simulink model "FOC_Motor_Tuning"  (R2025b)
settings: Solver=VariableStepAuto  StartTime=0.0  StopTime=8  RelTol=1e-3
values from neighbouring files (symbols this model uses):
  adc : value not decoded    [FoCFpgaData.sldd]
  dataRange = 800.0    [FoCFpgaData.sldd]
  encoder = 0.0    [FoCFpgaData.sldd]
  inverter = 24.0    [FoCFpgaData.sldd]
  paramAdcAmperePerCount : value not decoded    [FoCFpgaData.sldd]
  paramAdcCalibrationSamples = 16.0    [FoCFpgaData.sldd]
  paramAdcCountAtZeroAmpere : value not decoded    [FoCFpgaData.sldd]
  paramAdcEnablecalibration = 1.0    [FoCFpgaData.sldd]
  paramCurrentControlSatVoltage = 13.856406460551021    [FoCFpgaData.sldd]
  paramEncoderCalibrationDuration = 0.2    [FoCFpgaData.sldd]
  paramEncoderCalibrationMaxError = 0.0012566370614359172    [FoCFpgaData.sldd]
  paramEncoderCalibrationVoltage = 2.0    [FoCFpgaData.sldd]
  paramEncoderRotorPositionAtZeroCount = 0.0    [FoCFpgaData.sldd]
  paramOpenLoopVelocityAcceleration = 40.0    [FoCFpgaData.sldd]
  paramOpenLoopVelocityToVoltsBias = 0.4    [FoCFpgaData.sldd]
  paramOpenLoopVelocityToVoltsScalar = 0.04    [FoCFpgaData.sldd]
  paramOverCurrentDuration = 0.05    [FoCFpgaData.sldd]
  paramOverCurrentEnable = 0.0    [FoCFpgaData.sldd]
  paramOverCurrentLimit = 10.45    [FoCFpgaData.sldd]
  paramPwmCompareAtZeroVolt = 500.0    [FoCFpgaData.sldd]
  paramPwmCompareMax = 1000.0    [FoCFpgaData.sldd]
  paramPwmComparePerVolt = 41.666666666666664    [FoCFpgaData.sldd]
  paramVelocityControlSatCurrent = 3.5    [FoCFpgaData.sldd]
  PI_params = 0.00048000000000000007    [FoCFpgaData.sldd]
  pmsm : value not decoded    [FoCFpgaData.sldd]
  pwm = 2.0E-8    [FoCFpgaData.sldd]
  sampleTime = 4.0E-5    [FoCFpgaData.sldd]
libraries: fl_lib x12, nesl_utility x12, mcbeeMathTransformLib x8, simulink x4, slpidlib x4, ee_lib x4, mcbpositiondecoderlib x3, mcbcontrolslib x3, mcbplantlib x1, autolibpmsmexterior x1, eeGeneralControl x1, SignalEditorBlockLib x1
(part 2 of 3)

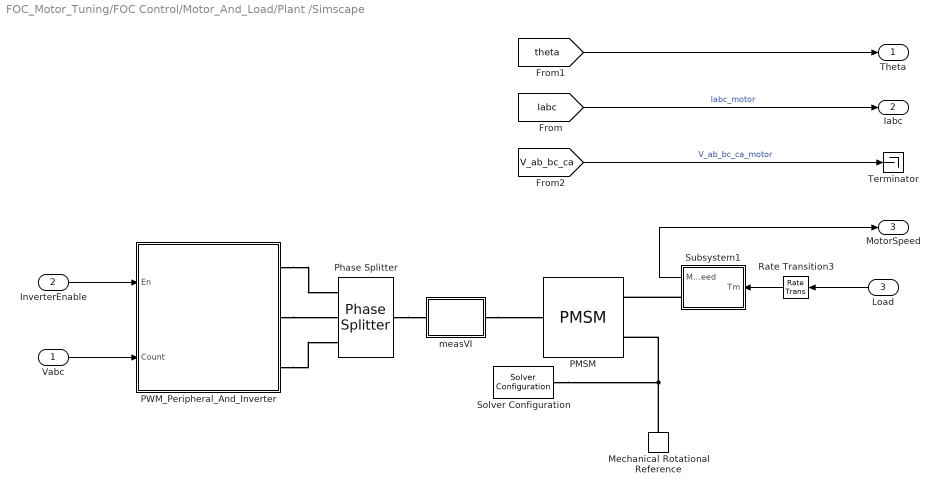
== system FOC_Motor_Tuning/FOC Control/Motor_And_Load/Plant /Simscape ==
  Vabc : Inport
  InverterEnable : Inport  Port=2
  Load : Inport  Port=3
  Mechanical Rotational Reference : fl_lib/Mechanical/Rotational Elements/Mechanical Rotational Reference
  PMSM : ee_lib/Electromechanical/Permanent Magnet/PMSM  port_option=ee.enum.threePhasePort.composite  winding_type=ee.enum.statorconnection.wye  machine_param=ee.enum.pmsm.parameterization.constant  nPolePairs=pmsm.p  pmflux_param=ee.enum.pmflux.fluxlinkage  pm_flux_linkage=pmsm.FluxPM Wb  torque_constant=0.18 N*m/A  back_emf_constant=0.18 V/(rad/s)  stator_param=ee.enum.statorparam.LdLqL0  Ld=pmsm.Ld H  Lq=pmsm.Lq H  idVec=[-200, 0, 200] A  iqVec=[-200, 0, 200] A  LdMatrix=0.0002 * ones(3, 3) H  LqMatrix=0.0002 * ones(3, 3) H  PmMatrix=0.1 * ones(3, 3) Wb  ktMatrix=0.18 * ones(3, 3) N*m/A  keMatrix=0.18 * ones(3, 3) V/(rad/s)  L0=0 H  Ls=0.0002 H  Lm=-0.00002 H  Ms=0.00002 H  Rs=pmsm.Rs Ohm  zero_sequence=ee.enum.park.zerosequence.exclude  axes_param=ee.enum.rotorangle.daxis  loss_param=ee.enum.ironloss.none  losses_oc=[0, 0, 0] W  losses_sc=[0, 0, 0] W  f_losses=60 Hz  Isc_losses=95 A  J=pmsm.J kg*m^2  lam=pmsm.B N*m/(rad/s)  i_d_specify=off  i_d_priority=None  i_d=0 A  i_d_nominal_specify=off  i_d_nominal_value=1  i_d_nominal_unit=A  i_q_specify=off  i_q_priority=None  i_q=0 A  i_q_nominal_specify=off  i_q_nominal_value=1  i_q_nominal_unit=A  torque_specify=off  torque_priority=None  torque=0 N*m  torque_nominal_specify=off  torque_nominal_value=1  torque_nominal_unit=N*m  angular_velocity_specify=off  angular_velocity_priority=High  angular_velocity=0 rpm  angular_velocity_nominal_specify=off  angular_velocity_nominal_value=1  angular_velocity_nominal_unit=rpm  angular_position_specify=off  angular_position_priority=High  angular_position=0 deg  angular_position_nominal_specify=off  angular_position_nominal_value=1  angular_position_nominal_unit=deg  alpha=3.93e-3 1/K  alpha_flux=-0.001 1/K  Tmeas=298.15 K  stator_thermal_mass=100 J/K  rotor_thermal_mass=200 J/K  Rm_percent_rotor=90  Rd_percent_rotor=30  temperatureA_specify=off  temperatureA_priority=High  temperatureA=25 degC  temperatureA_nominal_specify=off  temperatureA_nominal_value=1  temperatureA_nominal_unit=degC  temperatureB_specify=off  temperatureB_priority=High  temperatureB=25 degC  temperatureB_nominal_specify=off  temperatureB_nominal_value=1  temperatureB_nominal_unit=degC  temperatureC_specify=off  temperatureC_priority=High  temperatureC=25 degC  temperatureC_nominal_specify=off  temperatureC_nominal_value=1  temperatureC_nominal_unit=degC  temperatureR_specify=off  temperatureR_priority=High  temperatureR=25 degC  temperatureR_nominal_specify=off  temperatureR_nominal_value=1  temperatureR_nominal_unit=degC
      settings: InternalSimscapePortConfiguration="{\"Bottom\":[],\"Left\":[{\"id\":\"N\",\"label\":\"~\",\"type\":\"foundation.electrical.three_phase\"}],\"Right\":[{\"id\":\"R\",\"label\":\"R\",\"type\":\"foundation.mechanical.rotational.rotational\"},{\"id\":\"C\",\"label\":\"C\",\"type\":\"foundation.mechanical.rotational.rotational\"}],\"Top\":[]}"
  PWM_Peripheral_And_Inverter : Subsystem  VariantControl=variantPwm == enumPwm.behavior
      mask Display:
      | image('pwmPeripheralAndInverterMask.png')
      | port_label('input',1,'En')
      | port_label('input',2,'Compare')
      | text(0.98, 0.64, 'A', 'HorizontalAlignment', 'Right')
      | text(0.98, 0.38, 'B', 'HorizontalAlignment', 'Right')
      | text(0.98, 0.12, 'C', 'HorizontalAlignment', 'Right')
  Phase Splitter : ee_lib/Connectors & References/Phase Splitter
  Rate Transition3 : RateTransition  Deterministic=off  OutPortSampleTime=sampleTime.CurrentControl/2
  Solver Configuration : nesl_utility/Solver Configuration  PhysicalDomain=network_engine_domain  SubClassName=solver  LeftPortType=input  RightPortType=generic  Tones=[]  Harmonics=[]  SimulateNoise=off  Profile=off  UseLocalSampling=off  EnableSwitchedLinearOptims=on  FrequencyDomain=off  UseCCode=off  RelTol=0.001  AbsTol=1e-06  MinStep=1e-09  ToWorkspace=off  RevertToSquareIcSolve=off  NumHomotopyIterations=100  PhasorMode=off  PhasorModeNumHarmonics=1  ConsistencySolver=NEWTON_FTOL  IndexReductionMethod=DerivativeReplacement  DoDC=off  ResidualTolerance=1e-09  ConsistencyTolSource=GLOBAL  ConsistencyAbsTol=0.001  ConsistencyRelTol=0.001  ConsistencyTolFactor=0.001  UseLocalSolver=on  LocalSolverChoice=NE_BACKWARD_EULER_ADVANCER  ResolveIndetEquations=on  FunctionEvalNumThread=1  LocalSolverSampleTime=sampleTime.CurrentControl/2  DoFixedCost=on  MaxNonlinIter=3  MaxModeIter=2  ComputeImpulses=off  ImpulseIterations=1  LinearAlgebra=Full  LinearAlgebraNumThread=0  EquationFormulation=NE_TIME_EF  DelaysMemoryBudget=1024  AutomaticFiltering=off  FilteringTimeConstant=0.001  PartitionStorageMethod=AS_NEEDED  PartitionMemoryBudget=1024  PartitionMethod=ROBUST  MultibodyUseLocalSolver=off  MultibodyLocalSolverChoice=ODE1  MultibodyLocalSolverSampleTime=0.001
  Subsystem1 : Subsystem
  Terminator : Terminator
  measVI : Subsystem
  Theta : Outport
  Iabc : Outport  Port=2
  MotorSpeed : Outport  Port=3
  wires:
  Subsystem1/1(MotorSpeed) -> MotorSpeed/1
  [V_ab_bc_ca] -> Terminator/1  "V_ab_bc_ca_motor"
  Rate Transition3/1 -> Subsystem1/1(Tm)
  [theta] -> Theta/1
  [Iabc] -> Iabc/1  "Iabc_motor"
  Load/1 -> Rate Transition3/1
  Vabc/1 -> PWM_Peripheral_And_Inverter/2(Count)
  InverterEnable/1 -> PWM_Peripheral_And_Inverter/1(En)
  connections:
  Subsystem1/RConn1 -- PMSM/RConn1
  Mechanical Rotational Reference/LConn1 -- PMSM/RConn2 -- Solver Configuration/RConn1
  measVI/RConn1 -- PMSM/LConn1
  Phase Splitter/LConn1 -- measVI/LConn1
  PWM_Peripheral_And_Inverter/RConn1 -- Phase Splitter/RConn1
  PWM_Peripheral_And_Inverter/RConn2 -- Phase Splitter/RConn2
  PWM_Peripheral_And_Inverter/RConn3 -- Phase Splitter/RConn3

== system FOC_Motor_Tuning/FOC Control/Motor_And_Load/Sensor_Measurements/Get_PU  ==
  rad : Inport
  Constant2 : Constant  Value=2*pi  OutDataTypeStr=single  SampleTime=-1
  Get_PU : Gain  Gain=1/(2*pi)  RndMeth=Simplest  OutDataTypeStr=Inherit: Same as input
  Mod : Math  Operator=mod
  PU : Outport  VectorParamsAs1DForOutWhenUnconnected=off
  wires:
  rad/1 -> Mod/1
  Constant2/1 -> Mod/2
  Mod/1 -> Get_PU/1
  Get_PU/1 -> PU/1

== system FOC_Motor_Tuning/FOC Control/Motor_And_Load/Sensor_Measurements/Wrap ==
  in : Inport
  Constant2 : Constant  OutDataTypeStr=single  SampleTime=-1
  Mod : Math  Operator=mod
  out : Outport  VectorParamsAs1DForOutWhenUnconnected=off
  wires:
  in/1 -> Mod/1
  Constant2/1 -> Mod/2
  Mod/1 -> out/1

== system FOC_Motor_Tuning/FOC Control/Controller_Algorithm_Local/Algorithm_HDL/FOC_Velocity_Encoder/ADC_Count_To_Current ==
  note: ADC Count to Current
  Count : Inport  OutMin=0  OutMax=2^16-1  OutDataTypeStr=uint16  LockScale=on
  ADC_Offsets : Inport  Port=2
  Add : Sum  Inputs=+-  OutDataTypeStr=int32  SaturateOnIntegerOverflow=on  LockScale=on
  Data_Type_Convert : DataTypeConversion  OutDataTypeStr=int32  SaturateOnIntegerOverflow=off  RndMeth=Floor  LockScale=on
  Data_Type_Convert1 : DataTypeConversion  OutDataTypeStr=int32  SaturateOnIntegerOverflow=off  RndMeth=Floor  LockScale=on
  Product : Product  OutDataTypeStr=fixdt(1,32,19)
  Sat : Saturate  UpperLimit=dataRange.PhaseCurrent.Max  LowerLimit=dataRange.PhaseCurrent.Min  OutDataTypeStr=fixdt(1,16,11)
      settings: AttributesFormatString=-----------------\nLower = %<LowerLimit>\nUpper = %<UpperLimit>
  Scalar : Constant  Value=paramAdcAmperePerCount  OutDataTypeStr=fixdt(1,16,19)  SampleTime=-1
  Current : Outport  VectorParamsAs1DForOutWhenUnconnected=off
  ADC_Counts : Outport  Port=2  VectorParamsAs1DForOutWhenUnconnected=off
  wires:
  ADC_Offsets/1 -> Data_Type_Convert1/1
  Scalar/1 -> Product/2
  Add/1 -> Product/1
  Count/1 -> ADC_Counts/1, Data_Type_Convert/1
  Data_Type_Convert/1 -> Add/1
  Product/1 -> Sat/1
  Sat/1 -> Current/1
  Data_Type_Convert1/1 -> Add/2

== system FOC_Motor_Tuning/FOC Control/Controller_Algorithm_Local/Algorithm_HDL/FOC_Velocity_Encoder/Encoder_To_Position_And_Velocity ==
  note: Encoder To Position And Velocity
  Index_Found : Inport  OutDataTypeStr=boolean
  Count : Inport  Port=2  SampleTime=sampleTime.EncoderPosition
  Offset : Inport  Port=3  OutDataTypeStr=fixdt(1,16,12)  SampleTime=sampleTime.EncoderPosition
  Gain : Gain  Gain=2*pi  OutDataTypeStr=Inherit: Same as input
  Gain1 : Gain  Gain=1/(2*pi)  OutDataTypeStr=fixdt(1,16,12)
  Gain2 : Gain  Gain=2*pi  OutDataTypeStr=Inherit: Same as input
  Mechanical to Electrical Position : mcbpositiondecoderlib/Mechanical to Electrical Position  PolePairsInputType=Specify via dialog  NrPP=4  selectedRange=Per unit  MechOfstInputType=Input port  mechOffsetIn=0  maxAngleIn=1  InputDataType=fixdt(1,16,12)  VariantSelect=floating-point
  Quadrature Decoder : mcbpositiondecoderlib/Quadrature Decoder  ParameterInputType=off  CountsPerRevInverseDataType=single  EncoderSlitsPerRevolution=1250  EncoderCountsPerSlit=4  CounterSize=16 bits  ExternalIndexCount=off  PositionUnit=Per unit  PositionDataType=fixdt(1,16,12)
  Rotor_Position_Valid : Subsystem
  Speed Measurement : mcbpositiondecoderlib/Speed Measurement  DiscreteStepInput=off  LastDiscreteStepInput=off  PositionUnit=Per unit  PositionScalingDatatype=uint32  SpeedCalculationMode=Time interval for speed calculation  TempSpeedCalculationMode=Time interval for speed calculation  SampleTimeAsync=sampleTime.EncoderPosition  MaximumApplicationSpeed=4000  SpeedResolution=5e-6  DelayLength=30  MaximumMeasurableSpeed=24193.5484  MeasurableSpeedResolution=1.1642e-05  SpeedUnit=Radians/Sec  TempSpeedUnit=RPM  PerUnitSpeed=4000  SpeedDataType=fixdt(1,16,5)
  Rotor_Position : Outport  VectorParamsAs1DForOutWhenUnconnected=off
  Electrical_Position : Outport  Port=2  VectorParamsAs1DForOutWhenUnconnected=off
  Rotor_Velocity : Outport  Port=3  VectorParamsAs1DForOutWhenUnconnected=off
  wires:
  Offset/1 -> Rotor_Position_Valid/2(Encoder_Offset), Gain1/1  "offset"
  Mechanical to Electrical Position/1 -> Gain/1
  Gain/1 -> Electrical_Position/1  "radians"
  Quadrature Decoder/1 -> Gain2/1, Rotor_Position_Valid/1(Rotor_Position), Mechanical to Electrical Position/1
  Gain1/1 -> Mechanical to Electrical Position/2  "pu"
  Gain2/1 -> Rotor_Position/1  "rads"
  Speed Measurement/1 -> Rotor_Velocity/1
  Index_Found/1 -> Rotor_Position_Valid/3(Encoder_Index_Found)
  Count/1 -> Quadrature Decoder/1
  Rotor_Position_Valid/1(Position_Delta) -> Speed Measurement/1  "rotorPositionDelta"

== system FOC_Motor_Tuning/FOC Control/Controller_Algorithm_Local/Algorithm_HDL/FOC_Velocity_Encoder/FOC_Current_Control ==
  Reset : Inport
  Current_Command : Inport  Port=2  OutDataTypeStr=fixdt(1,16,11)
  Phase_Current : Inport  Port=3
  Electrical_Position : Inport  Port=4
  FOC_Current_Control_Fixdt : Subsystem  VariantControl=FixedPoint
  FOC_Current_Control_Single : Subsystem  VariantControl=FloatingPoint
  Phase_Voltage : Outport

== system FOC_Motor_Tuning/FOC Control/Controller_Algorithm_Local/Algorithm_HDL/FOC_Velocity_Encoder/Over_Current_Detector ==
  note: Over Current Detector
  Motor_On : Inport  OutMin=0  OutMax=1  OutDataTypeStr=boolean  LockScale=on
  Phase_Current : Inport  Port=2  OutMin=dataRange.PhaseCurrent.Min  OutMax=dataRange.PhaseCurrent.Max  OutDataTypeStr=fixdt(1,16,11)
  AND : Logic  IconShape=distinctive  AllPortsSameDT=off  OutDataTypeStr=boolean
  AND1 : Logic  IconShape=distinctive  AllPortsSameDT=off  OutDataTypeStr=boolean
  Abs : Abs  SaturateOnIntegerOverflow=off
      settings: LockScale=on
  Demux : Demux  Outputs=2
  Detect_Over_Current_Error : Stateflow chart  TreatAsAtomicUnit=on
  Enable_Over_Current_Detection : Constant  Value=paramOverCurrentEnable  OutDataTypeStr=boolean  SampleTime=-1  LockScale=on
  Motor_On1 : InportShadow  OutMin=0  OutMax=1  OutDataTypeStr=boolean
      settings: LockScale=on
  NOT : Logic  Operator=NOT  IconShape=distinctive  AllPortsSameDT=off  OutDataTypeStr=boolean
  Over_Current_Duration : Constant  Value=paramOverCurrentDuration  OutDataTypeStr=fixdt(1,16,14)  SampleTime=-1
  Over_Current_Limit : Constant  Value=paramOverCurrentLimit  OutDataTypeStr=fixdt(1,16,11)  SampleTime=-1
  Tick_Per_Sec : Gain  Gain=1/sampleTime.OverCurrentDetector  ParamDataTypeStr=fixdt(1,16,0)  OutDataTypeStr=uint16  LockScale=on
      settings: AttributesFormatString=---------------------------\nGain = %<Gain>
  En_Inv : Outport  VectorParamsAs1DForOutWhenUnconnected=off
  Error : Outport  Port=2  VectorParamsAs1DForOutWhenUnconnected=off
  wires:
  Tick_Per_Sec/1 -> Detect_Over_Current_Error/5(overCurrentDurationTicks)
  Phase_Current/1 -> Abs/1
  Abs/1 -> Demux/1
  Demux/2 -> Detect_Over_Current_Error/3(phaseCurrentB)
  Detect_Over_Current_Error/1(error) -> Error/1, NOT/1  "overCurrentErrorDetected"
  Over_Current_Duration/1 -> Tick_Per_Sec/1
  Over_Current_Limit/1 -> Detect_Over_Current_Error/4(overCurrentLimit)
  Demux/1 -> Detect_Over_Current_Error/2(phaseCurrentA)
  Motor_On/1 -> AND/1
  AND1/1 -> En_Inv/1  "enableInverter"
  NOT/1 -> AND1/2
  Motor_On1/1 -> AND1/1
  AND/1 -> Detect_Over_Current_Error/1(enableOverCurrentDetect)
  Enable_Over_Current_Detection/1 -> AND/2

== system FOC_Motor_Tuning/FOC Control/Controller_Algorithm_Local/Algorithm_HDL/FOC_Velocity_Encoder/Voltage_To_PWM_Compare ==
  note: Voltage To PWM Compare
  Voltage : Inport  OutMin=dataRange.PhaseVoltage.Min  OutMax=dataRange.PhaseVoltage.Max  OutDataTypeStr=fixdt(1,16,11)
  Add : Sum  OutDataTypeStr=fixdt(1,32,17)
  Bias : Constant  Value=paramPwmCompareAtZeroVolt  OutDataTypeStr=fixdt(1,16,2)  SampleTime=-1
  Data_Type_Conversion : DataTypeConversion  OutDataTypeStr=uint16  SaturateOnIntegerOverflow=off  RndMeth=Floor  LockScale=on
  Saturation : Saturate  UpperLimit=paramPwmCompareMax  LowerLimit=0
      settings: AttributesFormatString=|
      | --------------------------------
      | Upper Limit = %<UpperLimit>
      | Lower Limit = %<LowerLimit>
  Slope : Gain  Gain=paramPwmComparePerVolt  ParamDataTypeStr=fixdt(1,16,6)  OutDataTypeStr=fixdt(1,32,18)
      settings: AttributesFormatString=|
      | ----------------------------------------
      | Gain = %<Gain>
  Compare : Outport  VectorParamsAs1DForOutWhenUnconnected=off
  wires:
  Data_Type_Conversion/1 -> Compare/1  "pwmCompare"
  Voltage/1 -> Slope/1  "phaseVoltage"
  Slope/1 -> Add/1
  Saturation/1 -> Data_Type_Conversion/1
  Bias/1 -> Add/2
  Add/1 -> Saturation/1

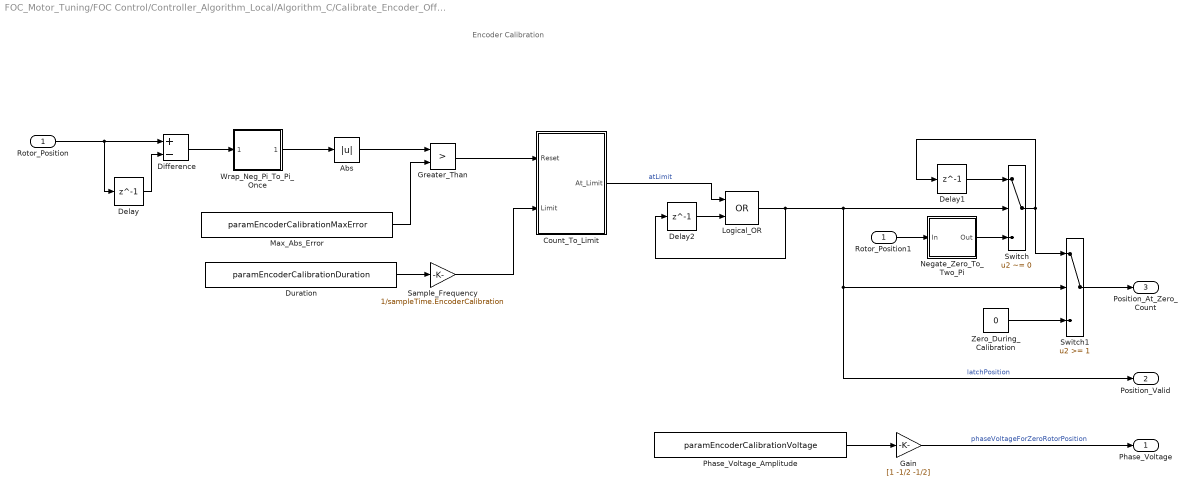
== system FOC_Motor_Tuning/FOC Control/Controller_Algorithm_Local/Algorithm_С/Calibrate_Encoder_Offset/Encoder_Calibration ==
  note: Encoder Calibration
  Rotor_Position : Inport  OutMin=0  OutMax=2*pi  PortDimensions=1  SampleTime=sampleTime.EncoderCalibration  Interpolate=off
  Abs : Abs  SaturateOnIntegerOverflow=off
  Count_To_Limit : Subsystem
  Delay : Delay  DelayLength=1
  Delay1 : Delay  DelayLength=1  InitialCondition=0
  Delay2 : Delay  DelayLength=1  InitialCondition=0
  Difference : Sum  Inputs=+-
  Duration : Constant  Value=paramEncoderCalibrationDuration  OutDataTypeStr=Inherit: Inherit via back propagation  SampleTime=-1
  Gain : Gain  Gain=[1 -1/2 -1/2]
      settings: AttributesFormatString=|
      | ----------------------------------
      | Gain = %<Gain>
  Greater_Than : RelationalOperator  Operator=>  OutDataTypeStr=boolean  InputSameDT=off
  Logical_OR : Logic  Operator=OR  IconShape=distinctive  AllPortsSameDT=off  OutDataTypeStr=boolean
  Max_Abs_Error : Constant  Value=paramEncoderCalibrationMaxError  OutDataTypeStr=Inherit: Inherit via back propagation  SampleTime=-1
  Negate_Zero_To_Two_Pi : Subsystem
      mask Display:
      | text(0.5, 0.5,['Negate' sprintf('\n') '0 to 2\pi'],...
      |   'HorizontalAlignment', 'Center',...
      |   'VerticalAlignment', 'Middle',...
      |   'texmode', 'on');
  Phase_Voltage_Amplitude : Constant  Value=paramEncoderCalibrationVoltage  OutDataTypeStr=Inherit: Inherit via back propagation  SampleTime=-1
  Rotor_Position1 : InportShadow  OutMin=0  OutMax=2*pi  PortDimensions=1  SampleTime=sampleTime.EncoderCalibration  Interpolate=off
  Sample_Frequency : Gain  Gain=1/sampleTime.EncoderCalibration
      settings: AttributesFormatString=|
      | ----------------------------------
      | Gain = %<Gain>
  Switch : Switch  Criteria=u2 ~= 0  Threshold=1  SaturateOnIntegerOverflow=off  InputSameDT=off
  Switch1 : Switch  Threshold=1  SaturateOnIntegerOverflow=off  InputSameDT=off
  Wrap_Neg_Pi_To_Pi_Once : Subsystem
      mask Display:
      | text(0.5, 0.5,['  Wrap' sprintf('\n') '-\pi to \pi'],...
      |   'HorizontalAlignment', 'Center',...
      |   'VerticalAlignment', 'Middle',...
      |   'texmode', 'on');
  Zero_During_Calibration : Constant  Value=0  OutDataTypeStr=Inherit: Inherit via back propagation
  Phase_Voltage : Outport  SampleTime=sampleTime.EncoderCalibration  InitialOutput=0  VectorParamsAs1DForOutWhenUnconnected=off
  Position_Valid : Outport  Port=2  SampleTime=sampleTime.EncoderCalibration  InitialOutput=0  VectorParamsAs1DForOutWhenUnconnected=off
  Position_At_Zero_Count : Outport  Port=3  SampleTime=sampleTime.EncoderCalibration  InitialOutput=0  VectorParamsAs1DForOutWhenUnconnected=off
  wires:
  Greater_Than/1 -> Count_To_Limit/1(Reset)
  Gain/1 -> Phase_Voltage/1  "phaseVoltageForZeroRotorPosition"
  Phase_Voltage_Amplitude/1 -> Gain/1
  Duration/1 -> Sample_Frequency/1
  Difference/1 -> Wrap_Neg_Pi_To_Pi_Once/1(Position)
  Wrap_Neg_Pi_To_Pi_Once/1(Wrap) -> Abs/1
  Switch1/1 -> Position_At_Zero_Count/1
  Abs/1 -> Greater_Than/1
  Max_Abs_Error/1 -> Greater_Than/2
  Zero_During_Calibration/1 -> Switch1/3
  Logical_OR/1 -> Delay2/1, Position_Valid/1, Switch1/2, Switch/2  "latchPosition"
  Rotor_Position/1 -> Delay/1, Difference/1
  Switch/1 -> Switch1/1, Delay1/1
  Delay/1 -> Difference/2
  Rotor_Position1/1 -> Negate_Zero_To_Two_Pi/1(In)
  Delay1/1 -> Switch/1
  Negate_Zero_To_Two_Pi/1(Out) -> Switch/3
  Sample_Frequency/1 -> Count_To_Limit/2(Limit)
  Count_To_Limit/1(At_Limit) -> Logical_OR/1  "atLimit"
  Delay2/1 -> Logical_OR/2

== system FOC_Motor_Tuning/FOC Control/Controller_Algorithm_Local/Algorithm_С/Open_Loop_Velocity_Control/Open_Loop_Velocity_Control ==
  note: Open Loop Velocity Control
  Velocity_Command : Inport  SampleTime=sampleTime.OpenLoopVelocityControl
  Direct_Voltage : Constant  Value=0  OutDataTypeStr=Inherit: Inherit via back propagation
  Electrical_Velocity_To_Position : Subsystem
  Inverse_Clarke_Transform : Subsystem  VariantControl=INVERSE_CLARKE_TRANSFORM
      mask Display:
      | port_label('input',1,'\alpha','texmode', 'on')
      | port_label('input',2,'\beta','texmode', 'on')
      | port_label('output',1,'ABC')
  Inverse_Park_Transform : Subsystem
      mask Display:
      | port_label('input',1,'D')
      | port_label('input',2,'Q')
      | port_label('input',3,'Sin')
      | port_label('input',4,'Cos')
      | port_label('output',1,'\alpha','texmode', 'on')
      | port_label('output',2,'\beta','texmode', 'on')
  Ramp_Velocity : Subsystem
  Rotor_Velocity_To_Volts : Subsystem
  Sine_Cosine : Trigonometry  Operator=sincos
  Phase_Voltage : Outport  SampleTime=sampleTime.OpenLoopVelocityControl  VectorParamsAs1DForOutWhenUnconnected=off
  wires:
  Inverse_Clarke_Transform/1(ABC) -> Phase_Voltage/1
  Velocity_Command/1 -> Ramp_Velocity/1(Velocity_Command)
  Rotor_Velocity_To_Volts/1(V) -> Inverse_Park_Transform/2(Q)  "quadratureVoltage"
  Direct_Voltage/1 -> Inverse_Park_Transform/1(D)
  Inverse_Park_Transform/1(Alpha) -> Inverse_Clarke_Transform/1(Alpha)
  Inverse_Park_Transform/2(Beta) -> Inverse_Clarke_Transform/2(Beta)
  Ramp_Velocity/1(Rotor_Velocity) -> Rotor_Velocity_To_Volts/1(RV)
  Ramp_Velocity/2(Electrical_Velocity) -> Electrical_Velocity_To_Position/1(EV)
  Sine_Cosine/1 -> Inverse_Park_Transform/3(Sin_Coefficient)
  Sine_Cosine/2 -> Inverse_Park_Transform/4(Cos_Coefficient)
  Electrical_Velocity_To_Position/1(EP) -> Sine_Cosine/1

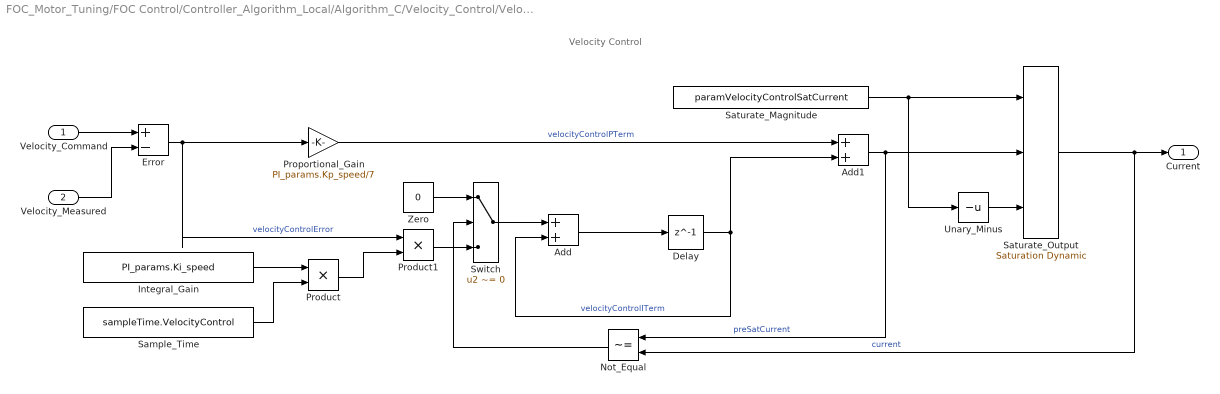
== system FOC_Motor_Tuning/FOC Control/Controller_Algorithm_Local/Algorithm_С/Velocity_Control/Velocity_Control ==
  note: Velocity Control
  Velocity_Command : Inport  SampleTime=sampleTime.VelocityControl
  Velocity_Measured : Inport  Port=2  SampleTime=sampleTime.VelocityControl
  Add : Sum
  Add1 : Sum
  Delay : Delay  DelayLength=1
  Error : Sum  Inputs=+-
  Integral_Gain : Constant  Value=PI_params.Ki_speed  OutDataTypeStr=Inherit: Inherit via back propagation
  Not_Equal : RelationalOperator  Operator=~=  OutDataTypeStr=boolean  InputSameDT=off
  Product : Product  OutDataTypeStr=Inherit: Same as first input
  Product1 : Product  OutDataTypeStr=Inherit: Same as first input
  Proportional_Gain : Gain  Gain=PI_params.Kp_speed/7
      settings: AttributesFormatString=|
      | -----------------------------------
      | Gain = %<Gain>
  Sample_Time : Constant  Value=sampleTime.VelocityControl  OutDataTypeStr=Inherit: Inherit via back propagation
  Saturate_Magnitude : Constant  Value=paramVelocityControlSatCurrent  OutDataTypeStr=Inherit: Inherit via back propagation
  Saturate_Output : simulink/Discontinuities/Saturation Dynamic  OutMin=[]  OutMax=[]  OutDataTypeStr=Inherit: Same as second input  OutDataType=fixdt(1, 16)  OutScaling=2^-10  DoSatur=off
  Switch : Switch  Criteria=u2 ~= 0  SaturateOnIntegerOverflow=off  InputSameDT=off
  Unary_Minus : UnaryMinus
  Zero : Constant  Value=0  OutDataTypeStr=Inherit: Inherit via back propagation
  Current : Outport  SampleTime=sampleTime.VelocityControl  VectorParamsAs1DForOutWhenUnconnected=off
  wires:
  Add/1 -> Delay/1
  Product1/1 -> Switch/3
  Product/1 -> Product1/2
  Sample_Time/1 -> Product/2
  Integral_Gain/1 -> Product/1
  Unary_Minus/1 -> Saturate_Output/3
  Saturate_Magnitude/1 -> Unary_Minus/1, Saturate_Output/1
  Zero/1 -> Switch/1
  Switch/1 -> Add/1
  Not_Equal/1 -> Switch/2
  Saturate_Output/1 -> Not_Equal/2, Current/1  "current"
  Error/1 -> Product1/1, Proportional_Gain/1  "velocityControlError"
  Proportional_Gain/1 -> Add1/1  "velocityControlPTerm"
  Velocity_Command/1 -> Error/1
  Add1/1 -> Saturate_Output/2, Not_Equal/1  "preSatCurrent"
  Delay/1 -> Add1/2, Add/2  "velocityControlITerm"
  Velocity_Measured/1 -> Error/2

== system FOC_Motor_Tuning/FOC Control/Motor_And_Load/Plant /MCB/Inverter ==
  Duty_abc : Inport
  Average-Value Inverter : mcbplantlib/Average-Value Inverter
  Constant2 : Constant  Value=inverter.V_dc  OutDataTypeStr=single  SampleTime=-1
  Data Type Conversion1 : DataTypeConversion  OutDataTypeStr=single  RndMeth=Simplest  SaturateOnIntegerOverflow=off
  Rate Transition3 : RateTransition  Deterministic=off  OutPortSampleTime=sampleTime.CurrentControl/2
  Vabc : Outport  VectorParamsAs1DForOutWhenUnconnected=off
  wires:
  Constant2/1 -> Average-Value Inverter/2
  Data Type Conversion1/1 -> Rate Transition3/1
  Duty_abc/1 -> Data Type Conversion1/1
  Rate Transition3/1 -> Average-Value Inverter/1
  Average-Value Inverter/1 -> Vabc/1

== system FOC_Motor_Tuning/FOC Control/Motor_And_Load/Plant /MCB/PWM_Count_to_Duty ==
  <pwmCompare> : Inport
  Add : Sum  Inputs=+-
  Bias : Constant  Value=paramPwmCompareAtZeroVolt  OutDataTypeStr=single  SampleTime=-1
  Constant : Constant  Value=0.5  OutDataTypeStr=single  SampleTime=-1
  Data Type Conversion : DataTypeConversion  OutDataTypeStr=single  SaturateOnIntegerOverflow=off  RndMeth=Floor
  Normalize [-0.5 to 0.5] : Gain  Gain=1/ (2 * inverter.V_dc / sqrt(3))  OutDataTypeStr=single  RndMeth=Simplest
  Slope : Gain  Gain=1/paramPwmComparePerVolt  ParamDataTypeStr=fixdt(1,16,6)  OutDataTypeStr=single
      settings: AttributesFormatString=|
      | ----------------------------------------
      | Gain = %<Gain>
  Sum : Sum  Inputs=|++
  Duty : Outport
  wires:
  Constant/1 -> Sum/2
  Normalize [-0.5 to 0.5]/1 -> Sum/1
  <pwmCompare>/1 -> Data Type Conversion/1
  Sum/1 -> Duty/1
  Data Type Conversion/1 -> Add/1
  Bias/1 -> Add/2
  Add/1 -> Slope/1
  Slope/1 -> Normalize [-0.5 to 0.5]/1

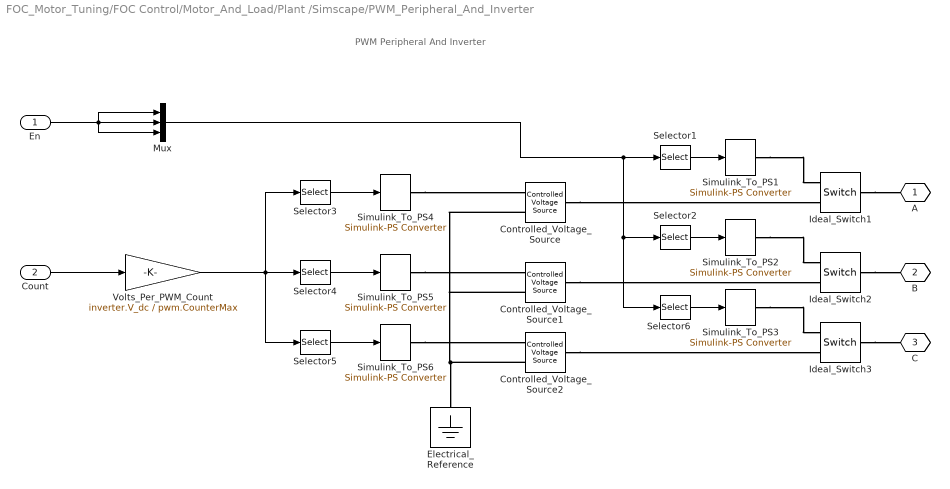
== system FOC_Motor_Tuning/FOC Control/Motor_And_Load/Plant /Simscape/PWM_Peripheral_And_Inverter ==
  note: PWM Peripheral And Inverter
  En : Inport
  Count : Inport  Port=2
  Controlled_Voltage_Source : fl_lib/Electrical/Electrical Sources/Controlled Voltage Source
  Controlled_Voltage_Source1 : fl_lib/Electrical/Electrical Sources/Controlled Voltage Source
  Controlled_Voltage_Source2 : fl_lib/Electrical/Electrical Sources/Controlled Voltage Source
  Electrical_Reference : fl_lib/Electrical/Electrical Elements/Electrical Reference
  Ideal_Switch1 : fl_lib/Electrical/Electrical Elements/Switch  R_closed=0.0001 Ohm  G_open=1e-5 1/Ohm  Threshold=0  i_specify=off  i_priority=None  i=0 A  i_nominal_specify=off  i_nominal_value=1  i_nominal_unit=A  v_specify=off  v_priority=None  v=0 V  v_nominal_specify=off  v_nominal_value=1  v_nominal_unit=V
  Ideal_Switch2 : fl_lib/Electrical/Electrical Elements/Switch  R_closed=0.0001 Ohm  G_open=1e-5 1/Ohm  Threshold=0  i_specify=off  i_priority=None  i=0 A  i_nominal_specify=off  i_nominal_value=1  i_nominal_unit=A  v_specify=off  v_priority=None  v=0 V  v_nominal_specify=off  v_nominal_value=1  v_nominal_unit=V
  Ideal_Switch3 : fl_lib/Electrical/Electrical Elements/Switch  R_closed=0.0001 Ohm  G_open=1e-5 1/Ohm  Threshold=0  i_specify=off  i_priority=None  i=0 A  i_nominal_specify=off  i_nominal_value=1  i_nominal_unit=A  v_specify=off  v_priority=None  v=0 V  v_nominal_specify=off  v_nominal_value=1  v_nominal_unit=V
  Mux : Mux  Inputs=3
  Selector1 : Selector  InputPortWidth=3  IndexOptions=Index vector (dialog)  Indices=[1]  OutputSizes=1
  Selector2 : Selector  InputPortWidth=3  IndexOptions=Index vector (dialog)  Indices=2  OutputSizes=1
  Selector3 : Selector  InputPortWidth=3  IndexOptions=Index vector (dialog)  Indices=[1]  OutputSizes=1
  Selector4 : Selector  InputPortWidth=3  IndexOptions=Index vector (dialog)  Indices=2  OutputSizes=1
  Selector5 : Selector  InputPortWidth=3  IndexOptions=Index vector (dialog)  Indices=3  OutputSizes=1
  Selector6 : Selector  InputPortWidth=3  IndexOptions=Index vector (dialog)  Indices=3  OutputSizes=1
  Simulink_To_PS{1..6} (6 alike) : nesl_utility/Simulink-PS Converter  PhysicalDomain=network_engine_domain  SubClassName=ps_input  LeftPortType=input  RightPortType=output  PseudoPeriodic=off  Frequencies=[]  NoiseDistribution=none  NoiseParameters=[]  Unit=1  AffineConversion=off  FilteringAndDerivatives=zero  SimscapeFilterOrder=1  InputFilterTimeConstant=0.001  UdotUserProvided=1
  Volts_Per_PWM_Count : Gain  Gain=inverter.V_dc / pwm.CounterMax  ParamDataTypeStr=double  OutDataTypeStr=double
      settings: AttributesFormatString=|
      | ----------------------------------------------------------------
      | Gain = %<Gain>
  A : PMIOPort  Tag=PMCPort  Side=Right
  B : PMIOPort  Tag=PMCPort  Port=2  Side=Right
  C : PMIOPort  Tag=PMCPort  Port=3  Side=Right
  wires:
  Selector1/1 -> Simulink_To_PS1/1
  Selector3/1 -> Simulink_To_PS4/1
  Selector4/1 -> Simulink_To_PS5/1
  Selector5/1 -> Simulink_To_PS6/1
  Volts_Per_PWM_Count/1 -> Selector5/1, Selector3/1, Selector4/1
  Count/1 -> Volts_Per_PWM_Count/1
  Selector2/1 -> Simulink_To_PS2/1
  Selector6/1 -> Simulink_To_PS3/1
  En/1 -> Mux/3, Mux/2, Mux/1
  Mux/1 -> Selector6/1, Selector2/1, Selector1/1
  connections:
  Ideal_Switch1/LConn1 -- A/RConn1
  Ideal_Switch2/LConn1 -- B/RConn1
  Ideal_Switch3/LConn1 -- C/RConn1
  Simulink_To_PS1/RConn1 -- Ideal_Switch1/RConn1
  Simulink_To_PS2/RConn1 -- Ideal_Switch2/RConn1
  Simulink_To_PS3/RConn1 -- Ideal_Switch3/RConn1
  Simulink_To_PS4/RConn1 -- Controlled_Voltage_Source/RConn1
  Controlled_Voltage_Source/LConn1 -- Ideal_Switch1/RConn2
  Controlled_Voltage_Source1/LConn1 -- Ideal_Switch2/RConn2
  Controlled_Voltage_Source2/LConn1 -- Ideal_Switch3/RConn2
  Simulink_To_PS6/RConn1 -- Controlled_Voltage_Source2/RConn1
  Simulink_To_PS5/RConn1 -- Controlled_Voltage_Source1/RConn1
  Controlled_Voltage_Source2/RConn2 -- Controlled_Voltage_Source/RConn2 -- Controlled_Voltage_Source1/RConn2 -- Electrical_Reference/LConn1

== system FOC_Motor_Tuning/FOC Control/Motor_And_Load/Plant /Simscape/Subsystem1 ==
  Tm : Inport
  Data Type Conversion1 : DataTypeConversion  SaturateOnIntegerOverflow=off  RndMeth=Floor
  Gain : Gain  Gain=2*pi/60
  Gain1 : Gain  Gain=-1
  Ideal Rotational Motion Sensor : fl_lib/Mechanical/Mechanical Sensors/Ideal Rotational Motion Sensor  reference=foundation.enum.MeasurementReference.difference  acceleration_port=false  velocity_port=true  position_port=true  wrap_angle=simscape.enum.onoff.off  offset=0 rad
  Ideal Torque Source : fl_lib/Mechanical/Mechanical Sources/Ideal Torque Source
  Mechanical Rotational Reference1 : fl_lib/Mechanical/Rotational Elements/Mechanical Rotational Reference
  Mechanical Rotational Reference2 : fl_lib/Mechanical/Rotational Elements/Mechanical Rotational Reference
  PS-Simulink Converter : nesl_utility/PS-Simulink Converter  PhysicalDomain=network_engine_domain  SubClassName=ps_output  LeftPortType=input  RightPortType=output  PseudoPeriodic=off  Frequencies=[]  VectorFormat=1-D array  Unit=rpm  AffineConversion=off
  PS-Simulink Converter1 : nesl_utility/PS-Simulink Converter  PhysicalDomain=network_engine_domain  SubClassName=ps_output  LeftPortType=input  RightPortType=output  PseudoPeriodic=off  Frequencies=[]  VectorFormat=1-D array  Unit=inherit  AffineConversion=off
  Rate Transition1 : RateTransition
  Simulink-PS Converter : nesl_utility/Simulink-PS Converter  PhysicalDomain=network_engine_domain  SubClassName=ps_input  LeftPortType=input  RightPortType=output  PseudoPeriodic=off  Frequencies=[]  NoiseDistribution=none  NoiseParameters=[]  Unit=N*m  AffineConversion=off  FilteringAndDerivatives=provide  SimscapeFilterOrder=1  InputFilterTimeConstant=0.001  UdotUserProvided=0
  "R " : PMIOPort  Side=Right
  MotorSpeed : Outport
  tag scope: theta=global
  wires:
  PS-Simulink Converter1/1 -> [theta]  "angle_motor"
  Gain/1 -> MotorSpeed/1  "speed_motor"
  PS-Simulink Converter/1 -> Gain/1
  Tm/1 -> Data Type Conversion1/1
  Data Type Conversion1/1 -> Gain1/1
  Rate Transition1/1 -> Simulink-PS Converter/1
  Gain1/1 -> Rate Transition1/1
  connections:
  Mechanical Rotational Reference2/LConn1 -- Ideal Rotational Motion Sensor/RConn1
  PS-Simulink Converter1/LConn1 -- Ideal Rotational Motion Sensor/RConn3
  Ideal Rotational Motion Sensor/RConn2 -- PS-Simulink Converter/LConn1
  "R "/RConn1 -- Ideal Rotational Motion Sensor/LConn1 -- Ideal Torque Source/LConn1
  Simulink-PS Converter/RConn1 -- Ideal Torque Source/RConn1
  Mechanical Rotational Reference1/LConn1 -- Ideal Torque Source/RConn2

== system FOC_Motor_Tuning/FOC Control/Motor_And_Load/Plant /Simscape/measVI ==
  Current Sensor (Three-Phase) : ee_lib/Sensors & Transducers/Current Sensor (Three-Phase)
  Line Voltage Sensor (Three-Phase) : ee_lib/Sensors & Transducers/Line Voltage Sensor (Three-Phase)
  Low-Pass Filter (Discrete or Continuous) : eeGeneralControl/Low-Pass Filter (Discrete or Continuous)  K=1  T=5e-4  B=inf  A=-inf  init_option=Inherited from block input  x0=0  Ts=-1
  PS-Simulink Converter2 : nesl_utility/PS-Simulink Converter  PhysicalDomain=network_engine_domain  SubClassName=ps_output  LeftPortType=input  RightPortType=output  PseudoPeriodic=off  Frequencies=[]  VectorFormat=1-D array  Unit=inherit  AffineConversion=off
  PS-Simulink Converter3 : nesl_utility/PS-Simulink Converter  PhysicalDomain=network_engine_domain  SubClassName=ps_output  LeftPortType=input  RightPortType=output  PseudoPeriodic=off  Frequencies=[]  VectorFormat=1-D array  Unit=inherit  AffineConversion=off
  ~1 : PMIOPort  Side=Left
  ~2 : PMIOPort  Port=2  Side=Right
  tag scope: Iabc=global, V_ab_bc_ca=global
  wires:
  Low-Pass Filter (Discrete or Continuous)/1 -> [V_ab_bc_ca]
  PS-Simulink Converter3/1 -> [Iabc]  "Iabc"
  PS-Simulink Converter2/1 -> Low-Pass Filter (Discrete or Continuous)/1  "Vabc"
  connections:
  Current Sensor (Three-Phase)/LConn1 -- ~1/RConn1 -- Line Voltage Sensor (Three-Phase)/LConn1
  Current Sensor (Three-Phase)/RConn2 -- ~2/RConn1
  PS-Simulink Converter2/LConn1 -- Line Voltage Sensor (Three-Phase)/RConn1
  Current Sensor (Three-Phase)/RConn1 -- PS-Simulink Converter3/LConn1

== system FOC_Motor_Tuning/FOC Control/Controller_Algorithm_Local/Algorithm_HDL/FOC_Velocity_Encoder/Encoder_To_Position_And_Velocity/Rotor_Position_Valid ==
  note: If offset changes, this is a bad sample since
      | the encoder was calibrated to a new value
  note: First two velocity calculations are not valid
  note: If detect positive rise in valid, this is a bad sample since
      | encoder index just reset
  note: Rotor Position Delta
  Rotor_Position : Inport  OutMin=0  OutMax=2*pi  OutDataTypeStr=fixdt(1,16,12)  SampleTime=sampleTime.EncoderPosition
  Encoder_Offset : Inport  Port=2  OutMin=-2*pi  OutMax=2*pi  OutDataTypeStr=fixdt(1,16,12)  SampleTime=sampleTime.EncoderPosition
  Encoder_Index_Found : Inport  Port=3  OutDataTypeStr=boolean  SampleTime=sampleTime.EncoderPosition  LockScale=on
  Constant : Constant  OutDataTypeStr=fixdt(1,16,14)  SampleTime=-1
  Delay1 : Delay  DelayLength=1
  Delay2 : Delay  DelayLength=1
  Delay3 : Delay  DelayLength=1
  Detect_Change : simulink/Logic and Bit Operations/Detect Change  vinit=0  OutDataTypeStr=boolean
  Detect_Rise : RelationalOperator  Operator=>  OutDataTypeStr=boolean  ZeroCross=off  InputSameDT=off
  Last_Valid_Position : Delay  DelayLength=1
  Logical_AND : Logic  Inputs=3  IconShape=distinctive  AllPortsSameDT=off  OutDataTypeStr=boolean
  No_Change_Detected : Logic  Operator=NOT  IconShape=distinctive  AllPortsSameDT=off  OutDataTypeStr=boolean
  No_Rise_Detected : Logic  Operator=NOT  IconShape=distinctive  AllPortsSameDT=off  OutDataTypeStr=boolean
  Switch : Switch  Criteria=u2 ~= 0  OutDataTypeStr=fixdt(1,16,12)  SaturateOnIntegerOverflow=off
  Position_Delta : Outport  SampleTime=sampleTime.EncoderPosition  VectorParamsAs1DForOutWhenUnconnected=off
  wires:
  Switch/1 -> Position_Delta/1, Last_Valid_Position/1
  No_Change_Detected/1 -> Logical_AND/2
  Detect_Change/1 -> No_Change_Detected/1
  Encoder_Offset/1 -> Detect_Change/1
  Rotor_Position/1 -> Switch/1
  Encoder_Index_Found/1 -> Detect_Rise/1, Delay3/1
  Delay2/1 -> Logical_AND/1
  Logical_AND/1 -> Switch/2  "positionDeltaValid"
  Delay3/1 -> Detect_Rise/2
  Last_Valid_Position/1 -> Switch/3
  Detect_Rise/1 -> No_Rise_Detected/1
  No_Rise_Detected/1 -> Logical_AND/3
  Constant/1 -> Delay1/1
  Delay1/1 -> Delay2/1

== system FOC_Motor_Tuning/FOC Control/Controller_Algorithm_Local/Algorithm_HDL/FOC_Velocity_Encoder/FOC_Current_Control/FOC_Current_Control_Fixdt ==
  note: FOC Current Control
  Reset : Inport  SampleTime=sampleTime.CurrentControl
  Current_Command : Inport  Port=2  OutMin=dataRange.PhaseCurrent.Min  OutMax=dataRange.PhaseCurrent.Max  OutDataTypeStr=fixdt(1,16,11)  SampleTime=sampleTime.CurrentControl
  Phase_Current : Inport  Port=3  OutMin=dataRange.PhaseCurrent.Min  OutMax=dataRange.PhaseCurrent.Max  OutDataTypeStr=fixdt(1,16,11)  SampleTime=sampleTime.CurrentControl
  Electrical_Position : Inport  Port=4  OutMin=0  OutMax=2*pi  OutDataTypeStr=fixdt(1,16,12)  SampleTime=sampleTime.CurrentControl
  Clarke Transform : mcbeeMathTransformLib/Clarke Transform  VariantControl=Variant2  PowerInvariant=off  UseWithEmbedded=on  PhaseInput=Two inputs
      settings: LibrarySourceBlock=mcbcontrolslib/Clarke Transform
  DQ_Current_Control : Subsystem
  Demux : Demux  Outputs=2
  Inverse Clarke Transform : mcbeeMathTransformLib/Inverse Clarke Transform  PowerInvariant=off  UseWithEmbedded=on  PhaseInput=Two inputs
      settings: LibrarySourceBlock=mcbcontrolslib/Inverse Clarke Transform
  Inverse Park Transform : mcbeeMathTransformLib/Park to Clarke Angle Transform  AxisAlignment=D-axis  UseWithEmbedded=on  PhaseInput=Two inputs  ThetaInput=Sine and Cosine electrical position  AngleInput=Per-unit  N_points=1024
      settings: LibrarySourceBlock=mcbcontrolslib/Inverse Park Transform
  Mux : Mux  Inputs=3
  PWM Reference Generator : mcbcontrolslib/PWM Reference Generator  inSignal=Vabc  modType=SVM: space vector modulation
      settings: LibrarySourceBlock=mcbhdllib/Controls/Math Transforms/PWM Reference Generator
  Park Transform : mcbeeMathTransformLib/Clarke to Park Angle Transform  AxisAlignment=D-axis  UseWithEmbedded=on  PhaseInput=Two inputs  ThetaInput=Sine and Cosine electrical position  AngleInput=Per-unit  N_points=1024
      settings: LibrarySourceBlock=mcbcontrolslib/Park Transform
  Sat : Saturate  UpperLimit=dataRange.PhaseVoltage.Max  LowerLimit=dataRange.PhaseVoltage.Min  OutDataTypeStr=fixdt(1,16,11)
      settings: AttributesFormatString=-----------------\nLower = %<LowerLimit>\nUpper = %<UpperLimit>
  Sine_Cosine : Subsystem
  Phase_Voltage : Outport  SampleTime=sampleTime.CurrentControl  VectorParamsAs1DForOutWhenUnconnected=off
  wires:
  Sine_Cosine/1(Sin) -> Inverse Park Transform/3, Park Transform/3  "sinCoefficient"
  Sine_Cosine/2(Cos) -> Inverse Park Transform/4, Park Transform/4  "cosCoefficient"
  Electrical_Position/1 -> Sine_Cosine/1(P)
  Phase_Current/1 -> Demux/1
  Clarke Transform/1 -> Park Transform/1  "alphaCurrent"
  Clarke Transform/2 -> Park Transform/2  "betaCurrent"
  Inverse Park Transform/1 -> Inverse Clarke Transform/1  "alphaVoltage"
  Inverse Park Transform/2 -> Inverse Clarke Transform/2  "betaVoltage"
  Park Transform/1 -> DQ_Current_Control/3(D_Current)  "dCurrent"
  Park Transform/2 -> DQ_Current_Control/4(Q_Current)  "qCurrent"
  Current_Command/1 -> DQ_Current_Control/2(Q_Command)
  DQ_Current_Control/1(D_Voltage) -> Inverse Park Transform/1  "dVoltage"
  DQ_Current_Control/2(Q_Voltage) -> Inverse Park Transform/2  "qVoltage"
  Mux/1 -> Sat/1  "svmVoltage"
  Sat/1 -> Phase_Voltage/1
  Reset/1 -> DQ_Current_Control/1(Reset)
  Demux/1 -> Clarke Transform/1
  Demux/2 -> Clarke Transform/2
  Inverse Clarke Transform/1 -> PWM Reference Generator/1
  Inverse Clarke Transform/2 -> PWM Reference Generator/2  "abcVoltage"
  Inverse Clarke Transform/3 -> PWM Reference Generator/3
  PWM Reference Generator/1 -> Mux/1
  PWM Reference Generator/2 -> Mux/2
  PWM Reference Generator/3 -> Mux/3

== system FOC_Motor_Tuning/FOC Control/Controller_Algorithm_Local/Algorithm_HDL/FOC_Velocity_Encoder/FOC_Current_Control/FOC_Current_Control_Single ==
  Reset : Inport
  Current_Command : Inport  Port=2
  Phase_Current : Inport  Port=3
  Electrical_Position : Inport  Port=4
  Data Type Conversion1 : DataTypeConversion  OutDataTypeStr=single  RndMeth=Nearest  SaturateOnIntegerOverflow=off
  Data Type Conversion2 : DataTypeConversion  OutDataTypeStr=single  RndMeth=Nearest  SaturateOnIntegerOverflow=off
  Data Type Conversion3 : DataTypeConversion  OutDataTypeStr=single  RndMeth=Nearest  SaturateOnIntegerOverflow=off
  Data Type Conversion4 : DataTypeConversion  OutDataTypeStr=fixdt(1,16,11)  RndMeth=Nearest  SaturateOnIntegerOverflow=off
  FOC_Current_Control : Subsystem
  Phase_Voltage : Outport  VectorParamsAs1DForOutWhenUnconnected=off
  wires:
  Current_Command/1 -> Data Type Conversion1/1
  Data Type Conversion3/1 -> FOC_Current_Control/4(Electrical_Position)
  FOC_Current_Control/1(Phase_Voltage) -> Data Type Conversion4/1
  Reset/1 -> FOC_Current_Control/1(Reset)
  Data Type Conversion1/1 -> FOC_Current_Control/2(Current_Command)
  Data Type Conversion2/1 -> FOC_Current_Control/3(Phase_Current)
  Electrical_Position/1 -> Data Type Conversion3/1
  Phase_Current/1 -> Data Type Conversion2/1
  Data Type Conversion4/1 -> Phase_Voltage/1

== system FOC_Motor_Tuning/FOC Control/Controller_Algorithm_Local/Algorithm_С/Calibrate_Encoder_Offset/Encoder_Calibration/Count_To_Limit ==
  note: Count To Limit
  Reset : Inport
  Limit : Inport  Port=2
  Add : Sum
  Continue_Count : Constant  OutDataTypeStr=Inherit: Inherit via back propagation
  Delay : Delay  DelayLength=1  InitialCondition=0
  Delay1 : Delay  DelayLength=1  InitialCondition=0
  Greater_Or_Equal : RelationalOperator  OutDataTypeStr=boolean  InputSameDT=off
  Reset_Count : Constant  Value=0  OutDataTypeStr=Inherit: Inherit via back propagation
  Stop_Count : Constant  Value=0  OutDataTypeStr=Inherit: Inherit via back propagation
  Switch : Switch  Threshold=1  SaturateOnIntegerOverflow=off  InputSameDT=off
  Switch1 : Switch  Threshold=1  SaturateOnIntegerOverflow=off  InputSameDT=off
  At_Limit : Outport  VectorParamsAs1DForOutWhenUnconnected=off
  wires:
  Add/1 -> Switch/3
  Reset_Count/1 -> Switch/1
  Reset/1 -> Switch/2
  Delay/1 -> Add/2
  Greater_Or_Equal/1 -> At_Limit/1, Delay1/1
  Stop_Count/1 -> Switch1/1
  Switch/1 -> Greater_Or_Equal/1, Delay/1
  Continue_Count/1 -> Switch1/3
  Switch1/1 -> Add/1
  Limit/1 -> Greater_Or_Equal/2
  Delay1/1 -> Switch1/2

== system FOC_Motor_Tuning/FOC Control/Controller_Algorithm_Local/Algorithm_С/Calibrate_Encoder_Offset/Encoder_Calibration/Negate_Zero_To_Two_Pi ==
  note: Negate Zero To Two Pi
  In : Inport
  Input_Range : SignalSpecification  OutMin=0  OutMax=2*pi
      settings: AttributesFormatString=|
      | -----------------------
      | Min = %<OutMin>
      | Max = %<OutMax>
  Subtract : Sum  Inputs=+-  OutDataTypeStr=Inherit: Inherit via back propagation
  Two_Pi : Constant  Value=2*pi  OutDataTypeStr=Inherit: Inherit via back propagation
  Out : Outport  VectorParamsAs1DForOutWhenUnconnected=off
  wires:
  Subtract/1 -> Out/1  "negativeIn"
  In/1 -> Input_Range/1
  Two_Pi/1 -> Subtract/1
  Input_Range/1 -> Subtract/2

== system FOC_Motor_Tuning/FOC Control/Controller_Algorithm_Local/Algorithm_С/Calibrate_Encoder_Offset/Encoder_Calibration/Wrap_Neg_Pi_To_Pi_Once ==
  note: Wrap Neg Pi To Pi Once
  Position : Inport
  Add : Sum  Inputs=+-  OutDataTypeStr=Inherit: Inherit via back propagation
  Add1 : Sum
  Greater_Than : RelationalOperator  OutDataTypeStr=boolean  InputSameDT=off
  Input_Range : SignalSpecification  OutMin=-4*pi  OutMax=4*pi
      settings: AttributesFormatString=|
      | -----------------------
      | Min = %<OutMin>
      | Max = %<OutMax>
  Less_Than : RelationalOperator  Operator=<  OutDataTypeStr=boolean  InputSameDT=off
  Neg_Pi : Constant  Value=-pi  OutDataTypeStr=Inherit: Inherit via back propagation
  Output_Range : SignalSpecification  OutMin=-pi  OutMax=pi
      settings: AttributesFormatString=|
      | -----------------------
      | Min = %<OutMin>
      | Max = %<OutMax>
  PI : Constant  Value=pi  OutDataTypeStr=Inherit: Inherit via back propagation
  Switch1 : Switch  Criteria=u2 ~= 0  SaturateOnIntegerOverflow=off  InputSameDT=off
  Switch2 : Switch  Criteria=u2 ~= 0  SaturateOnIntegerOverflow=off  InputSameDT=off
  Two_Pi : Constant  Value=2*pi  OutDataTypeStr=Inherit: Inherit via back propagation
  Two_Pi2 : Constant  Value=2*pi  OutDataTypeStr=Inherit: Inherit via back propagation
  Wrap : Outport  VectorParamsAs1DForOutWhenUnconnected=off
  wires:
  Position/1 -> Input_Range/1
  PI/1 -> Greater_Than/2
  Neg_Pi/1 -> Less_Than/2
  Greater_Than/1 -> Switch1/2  "positionGreaterThanPii"
  Two_Pi/1 -> Add/2
  Add/1 -> Switch1/1  "wrapPositionPi"
  Less_Than/1 -> Switch2/2  "positionLessThanPi"
  Switch2/1 -> Switch1/3
  Two_Pi2/1 -> Add1/2
  Add1/1 -> Switch2/1  "wrapPositionNegPii"
  Switch1/1 -> Output_Range/1
  Output_Range/1 -> Wrap/1
  Input_Range/1 -> Less_Than/1, Switch2/3, Add1/1, Add/1, Greater_Than/1

== system FOC_Motor_Tuning/FOC Control/Controller_Algorithm_Local/Algorithm_С/Open_Loop_Velocity_Control/Open_Loop_Velocity_Control/Electrical_Velocity_To_Position ==
  note: Electrical Velocity To Position
  EV : Inport
  Add : Sum
  Delay : Delay  DelayLength=1
  Gain : Gain  Gain=sampleTime.OpenLoopVelocityControl  OutDataTypeStr=Inherit: Inherit via back propagation
      settings: AttributesFormatString=------------------------------\nGain = %<Gain>
  Mod_Two_Pi_Once : Subsystem
      mask Display:
      | text(0.5, 0.5,'Mod 2\pi',...
      |   'HorizontalAlignment', 'Center',...
      |   'VerticalAlignment', 'Middle',...
      |   'texmode', 'on')
  EP : Outport  VectorParamsAs1DForOutWhenUnconnected=off
  wires:
  Delay/1 -> Add/2, EP/1
  Gain/1 -> Add/1
  EV/1 -> Gain/1
  Mod_Two_Pi_Once/1(Mod_X_Two_Pi) -> Delay/1
  Add/1 -> Mod_Two_Pi_Once/1(X)

== system FOC_Motor_Tuning/FOC Control/Controller_Algorithm_Local/Algorithm_С/Open_Loop_Velocity_Control/Open_Loop_Velocity_Control/Inverse_Clarke_Transform ==
  note: Inverse Clarke Transform
  note: Converts direct axis (alpha) component and the quadrature axis (beta) component to balanced three-phase quantities
      | The alpha and beta components are dependent on time and speed.
  Alpha : Inport
  Beta : Inport  Port=2
  Add : Sum  Inputs=-+  OutDataTypeStr=Inherit: Same as first input
  Add1 : Sum  Inputs=--  OutDataTypeStr=Inherit: Same as first input
  Gain : Gain  Gain=1/2
  Gain1 : Gain  Gain=sqrt(3)/2
  Mux : Mux  Inputs=3
  ABC : Outport  VectorParamsAs1DForOutWhenUnconnected=off
  wires:
  Gain/1 -> Add1/1, Add/1
  Gain1/1 -> Add1/2, Add/2
  Add/1 -> Mux/2
  Add1/1 -> Mux/3
  Beta/1 -> Gain1/1
  Alpha/1 -> Mux/1, Gain/1
  Mux/1 -> ABC/1
